simulink model "NonlinearSystemIdentificationMethod2"  (R2022b)
settings: Solver=VariableStepAuto  StartTime=0.0  StopTime=2.155  RelTol=1e-3
undefined symbols (not defined in the file): K, L, T
settings Model: Creator=amirz  LastModifiedBy=amirz

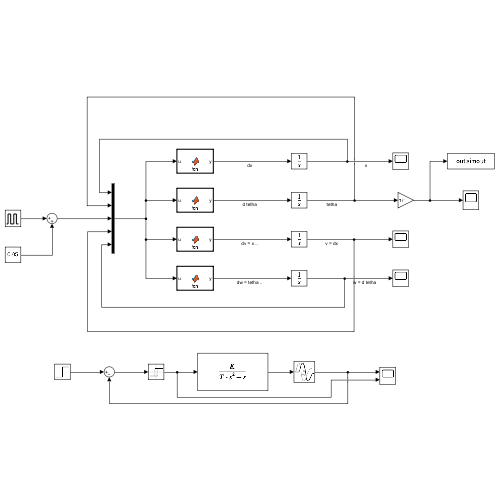
[thumbnail: Simulink's stored preview of the top-level diagram]
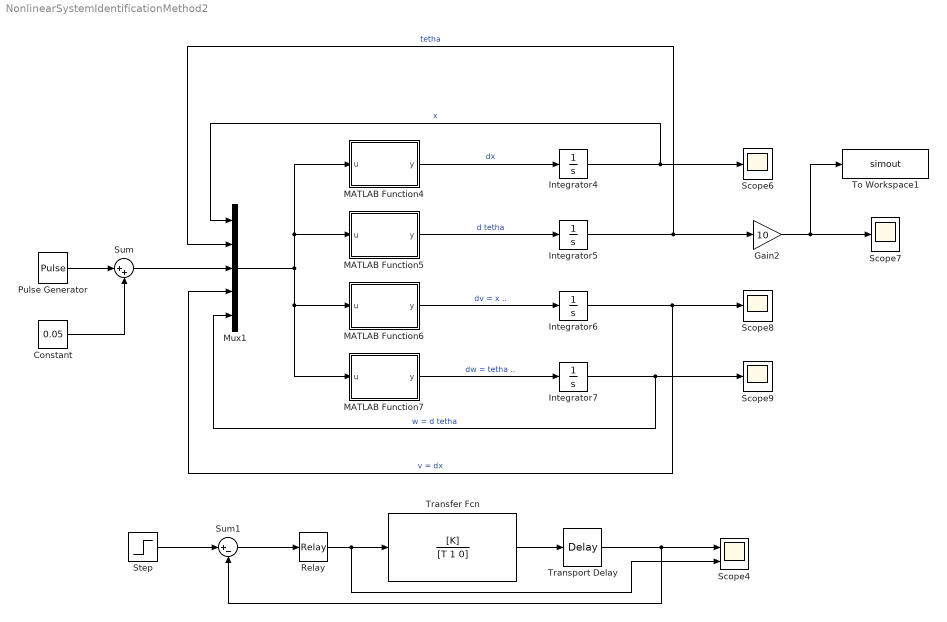
== system NonlinearSystemIdentificationMethod2 ==
  Constant : Constant  Value=0.05
  Gain2 : Gain  Gain=10
  Integrator{4..7} (4 alike) : Integrator
  MATLAB Function4 : MATLAB Function  TreatAsAtomicUnit=on
  MATLAB Function5 : MATLAB Function  TreatAsAtomicUnit=on
  MATLAB Function6 : MATLAB Function  TreatAsAtomicUnit=on
  MATLAB Function7 : MATLAB Function  TreatAsAtomicUnit=on
  Mux1 : Mux  Inputs=5
  Pulse Generator : DiscretePulseGenerator  PulseType=Time based  Amplitude=-0.1  Period=0.001  PulseWidth=50
  Relay : Relay  OffOutputValue=-1
  Scope4 : Scope  NumInputPorts=2
  Scope{6..9} (4 alike) : Scope
  Step : Step  Time=0  After=0  SampleTime=0
  Sum : Sum  Inputs=|++
  Sum1 : Sum  Inputs=|+-
  To Workspace1 : ToWorkspace  VariableName=simout  SaveFormat=Timeseries  SampleTime=-1
  Transfer Fcn : TransferFcn  Numerator=[K]  Denominator=[T 1 0]
  Transport Delay : TransportDelay  DelayTime=L
  wires:
  Transfer Fcn/1 -> Transport Delay/1
  Transport Delay/1 -> Scope4/1, Sum1/2
  Relay/1 -> Scope4/2, Transfer Fcn/1
  Sum1/1 -> Relay/1
  Step/1 -> Sum1/1
  Constant/1 -> Sum/2
  Pulse Generator/1 -> Sum/1
  Mux1/1 -> MATLAB Function6/1(u), MATLAB Function7/1(u), MATLAB Function4/1(u), MATLAB Function5/1(u)
  MATLAB Function5/1(y) -> Integrator5/1  "d tetha"
  MATLAB Function6/1(y) -> Integrator6/1  "dv = x .."
  Integrator6/1 -> Mux1/4, Scope8/1  "v = dx"
  Sum/1 -> Mux1/3
  MATLAB Function4/1(y) -> Integrator4/1  "dx"
  MATLAB Function7/1(y) -> Integrator7/1  "dw = tetha .."
  Integrator4/1 -> Mux1/1, Scope6/1  "x"
  Integrator5/1 -> Gain2/1, Mux1/2  "tetha"
  Integrator7/1 -> Mux1/5, Scope9/1  "w = d tetha"
  Gain2/1 -> To Workspace1/1, Scope7/1

== matlab function NonlinearSystemIdentificationMethod2/MATLAB Function5 ==
  data: u input size=[1,5]; y output
function y = fcn(u)
M = 10;
m = 0.3;
l = 0.3;
g = 9.8;
y = u(5);

== matlab function NonlinearSystemIdentificationMethod2/MATLAB Function6 ==
  data: u input size=[1,5]; y output
function y = fcn(u)
M = 10;
m = 0.3;
l = 0.3;
g = 9.8;
y = (u(3) + m*l*u(5)*u(5)*sin(u(2)) - m*g*sin(u(2))*cos(u(2)))/(M + m - m*cos(u(2))*cos(u(2)));

== matlab function NonlinearSystemIdentificationMethod2/MATLAB Function7 ==
  data: u input size=[1,5]; y output
function y = fcn(u)
M = 10;
m = 0.3;
l = 0.3;
g = 9.8;
y = (-u(3)*cos(u(2)) - m*l*u(5)*u(5)*sin(u(2))*cos(u(2)) + M*g*sin(u(2)) + m*g*sin(u(2)))/(l*M + l*m - l*m*cos(u(2))*cos(u(2)));

== matlab function NonlinearSystemIdentificationMethod2/MATLAB Function4 ==
  data: u input size=[1,5]; y output
function y = fcn(u)
M = 10;
m = 0.3;
l = 0.3;
g = 9.8;
y = u(4);
